simulink model "ALS"  (R2019b)
settings: Solver=ode1  StartTime=0.0  StopTime=200  FixedStep=0.05  RelTol=1e-3  EnableMultiTasking=on
undefined symbols (not defined in the file): ACSP
libraries: simulink x2
(part 2 of 2)

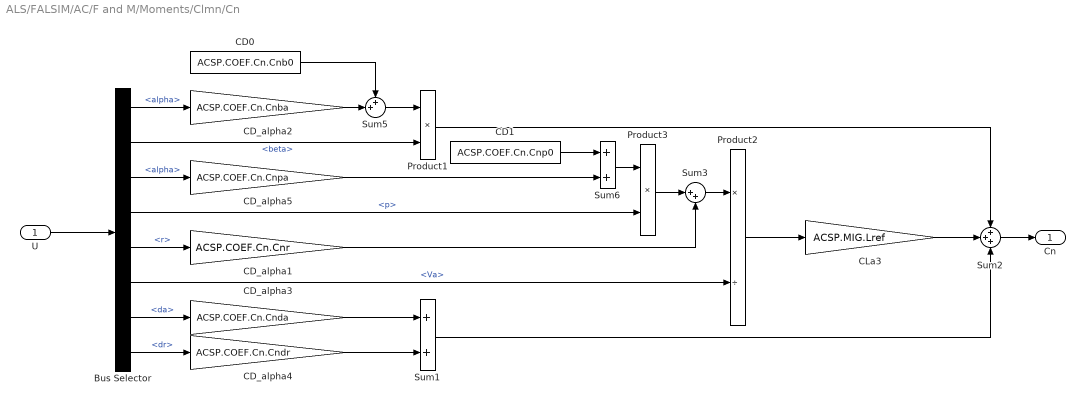
== system ALS/FALSIM/AC/F and M/Moments/Clmn/Cn ==
  U : Inport
  Bus Selector : BusSelector  OutputSignals=alpha,beta,alpha,p,r,Va,da,dr
  CD0 : Constant  Value=ACSP.COEF.Cn.Cnb0
  CD1 : Constant  Value=ACSP.COEF.Cn.Cnp0
  CD_alpha1 : Gain  Gain=ACSP.COEF.Cn.Cnr
  CD_alpha2 : Gain  Gain=ACSP.COEF.Cn.Cnba
  CD_alpha3 : Gain  Gain=ACSP.COEF.Cn.Cnda
  CD_alpha4 : Gain  Gain=ACSP.COEF.Cn.Cndr
  CD_alpha5 : Gain  Gain=ACSP.COEF.Cn.Cnpa
  CLa3 : Gain  Gain=ACSP.MIG.Lref
  Product1 : Product  RndMeth=Zero
  Product2 : Product  Inputs=*/  RndMeth=Zero
  Product3 : Product  RndMeth=Zero
  Sum1 : Sum
  Sum2 : Sum  Inputs=+++
  Sum3 : Sum  Inputs=|++
  Sum5 : Sum  Inputs=++|
  Sum6 : Sum
  Cn : Outport
  wires:
  U/1 -> Bus Selector/1
  Product2/1 -> CLa3/1
  Sum2/1 -> Cn/1
  Bus Selector/1 -> CD_alpha2/1  "<alpha>"
  CD_alpha2/1 -> Sum5/2
  CD0/1 -> Sum5/1
  Bus Selector/2 -> Product1/2  "<beta>"
  Sum5/1 -> Product1/1
  Bus Selector/3 -> CD_alpha5/1  "<alpha>"
  Product1/1 -> Sum2/1
  CD_alpha5/1 -> Sum6/2
  CD1/1 -> Sum6/1
  Sum6/1 -> Product3/1
  Bus Selector/4 -> Product3/2  "<p>"
  Bus Selector/5 -> CD_alpha1/1  "<r>"
  CD_alpha1/1 -> Sum3/2
  Bus Selector/6 -> Product2/2  "<Va>"
  Bus Selector/7 -> CD_alpha3/1  "<da>"
  Bus Selector/8 -> CD_alpha4/1  "<dr>"
  CD_alpha3/1 -> Sum1/1
  CD_alpha4/1 -> Sum1/2
  Sum1/1 -> Sum2/3
  CLa3/1 -> Sum2/2
  Product3/1 -> Sum3/1
  Sum3/1 -> Product2/1
